simulink model "model"  (R2024b)
settings: Solver=ode45  StartTime=0.0  StopTime=stop_time  RelTol=1e-3
undefined symbols (not defined in the file): controller, plant, reference
settings Model: Creator=sam  LastModifiedBy=sam

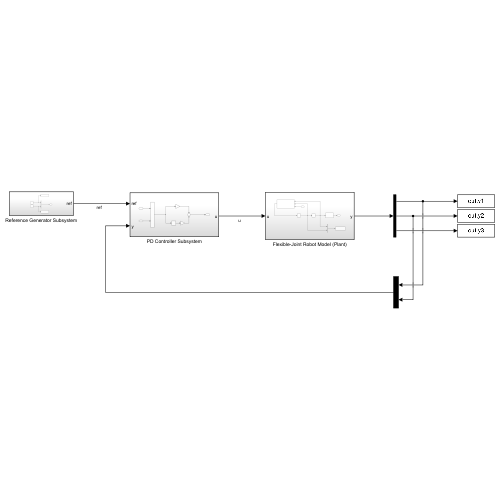
[thumbnail: Simulink's stored preview of the top-level diagram]
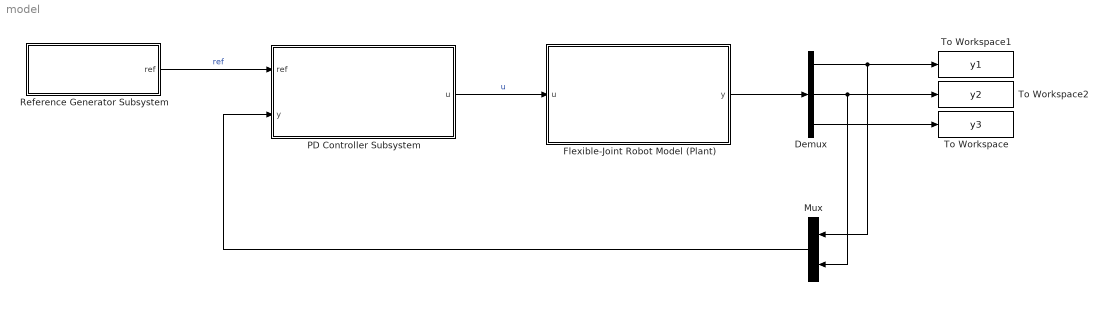
== system model ==
  Demux : Demux  Outputs=3
  Flexible-Joint Robot Model (Plant) : Subsystem
  Mux : Mux  Inputs=2
  PD Controller Subsystem : Subsystem
  Reference Generator Subsystem : Subsystem
  To Workspace : ToWorkspace  VariableName=y3  SaveFormat=Structure With Time  SampleTime=-1
  To Workspace1 : ToWorkspace  VariableName=y1  SaveFormat=Structure With Time  SampleTime=-1
  To Workspace2 : ToWorkspace  VariableName=y2  SaveFormat=Structure With Time  SampleTime=-1
  wires:
  Reference Generator Subsystem/1(ref) -> PD Controller Subsystem/1(ref)  "ref"
  PD Controller Subsystem/1(u) -> Flexible-Joint Robot Model (Plant)/1(u)  "u"
  Demux/3 -> To Workspace/1
  Flexible-Joint Robot Model (Plant)/1(y) -> Demux/1
  Mux/1 -> PD Controller Subsystem/2(y)
  Demux/2 -> To Workspace2/1, Mux/2
  Demux/1 -> To Workspace1/1, Mux/1

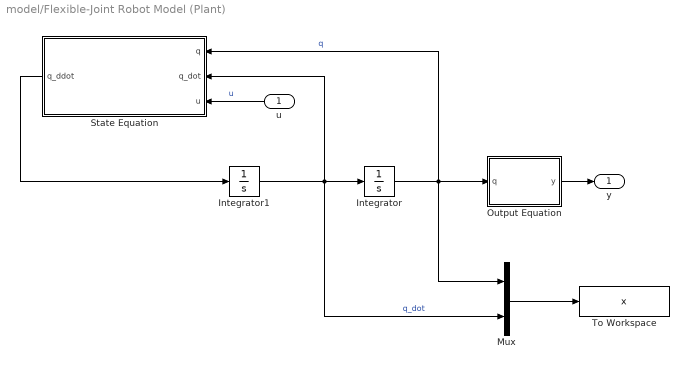
== system model/Flexible-Joint Robot Model (Plant) ==
  u : Inport
  Integrator : Integrator  InitialCondition=plant.initial.q
  Integrator1 : Integrator  InitialCondition=plant.initial.qdot
  Mux : Mux  Inputs=2
  Output Equation : MATLAB Function  TreatAsAtomicUnit=on
  State Equation : MATLAB Function  TreatAsAtomicUnit=on
  To Workspace : ToWorkspace  VariableName=x  SaveFormat=Structure With Time  SampleTime=-1
  y : Outport
  wires:
  Output Equation/1(y) -> y/1
  u/1 -> State Equation/3(u)  "u"
  Integrator1/1 -> Mux/2, State Equation/2(q_dot), Integrator/1  "q_dot"
  State Equation/1(q_ddot) -> Integrator1/1
  Integrator/1 -> Mux/1, State Equation/1(q), Output Equation/1(q)  "q"
  Mux/1 -> To Workspace/1

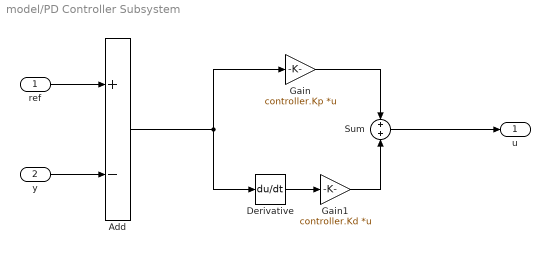
== system model/PD Controller Subsystem ==
  ref : Inport
  y : Inport  Port=2
  Add : Sum  Inputs=+-
  Derivative : Derivative
  Gain : Gain  Gain=controller.Kp  Multiplication=Matrix(K*u)
  Gain1 : Gain  Gain=controller.Kd  Multiplication=Matrix(K*u)
  Sum : Sum  Inputs=+|+
  u : Outport
  wires:
  Gain/1 -> Sum/1
  Sum/1 -> u/1
  Add/1 -> Derivative/1, Gain/1
  y/1 -> Add/2
  Derivative/1 -> Gain1/1
  ref/1 -> Add/1
  Gain1/1 -> Sum/2

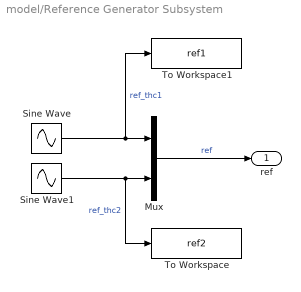
== system model/Reference Generator Subsystem ==
  Mux : Mux  Inputs=2
  Sine Wave : Sin  Amplitude=reference.thc1.A  Frequency=reference.thc1.w  SampleTime=0.001
  Sine Wave1 : Sin  Amplitude=reference.thc2.A  Frequency=reference.thc2.w  SampleTime=0.001
  To Workspace : ToWorkspace  VariableName=ref2  SaveFormat=Structure With Time  SampleTime=-1
  To Workspace1 : ToWorkspace  VariableName=ref1  SaveFormat=Structure With Time  SampleTime=-1
  ref : Outport
  wires:
  Mux/1 -> ref/1  "ref"
  Sine Wave/1 -> To Workspace1/1, Mux/1  "ref_thc1"
  Sine Wave1/1 -> To Workspace/1, Mux/2  "ref_thc2"

== matlab function model/Flexible-Joint Robot Model (Plant)/Output Equation ==
  data: q input; y output
function y = f_out_block(q)
% Call the CasADi function which models the output equation of the model.
% Input:
%   q : [4x1] [theta1; theta2; delta1; delta2]
% Output:
%   y : [3x1] [y1, y2, y3]

% Declare f_out as extrinsic
coder.extrinsic('f_out_mex');

% Allocate y variable
y = zeros(3,1);

% Call mex function built using CasADi
y = f_out_mex('f_out', q);
end

== matlab function model/Flexible-Joint Robot Model (Plant)/State Equation ==
  data: q input; q_ddot output; q_dot input; u input
function q_ddot = f_dyn_block(q, q_dot, u)
% Call the CasADi function which models the dynamics of the robot.
% Inputs:
%   q      : [4x1] [theta1; theta2; delta1; delta2]
%   q_dot  : [4x1] [dtheta1; dtheta2; ddelta1; ddelta2]
%   u      : [2x1] [u1; u2]
% Output:
%   q_ddot : [4x1] accelerations

% Declare f_dyn as extrinsic
coder.extrinsic('f_dyn_mex');

% Allocate q_ddot variable
q_ddot = zeros(4,1);

% Call mex function built using CasADi
q_ddot = f_dyn_mex('f_dyn', q, q_dot, u);

end
